simulink model "Hexapod_Robot_Leg"  (Simulink 8.3)
settings: Solver=ode45  StartTime=0.0  StopTime=inf  RelTol=1e-3
undefined symbols (not defined in the file): get, hot
libraries: mblibv1 x70, simulink_need_slupdate x18, vrlib x7, dspsnks4 x1
(part 2 of 2)

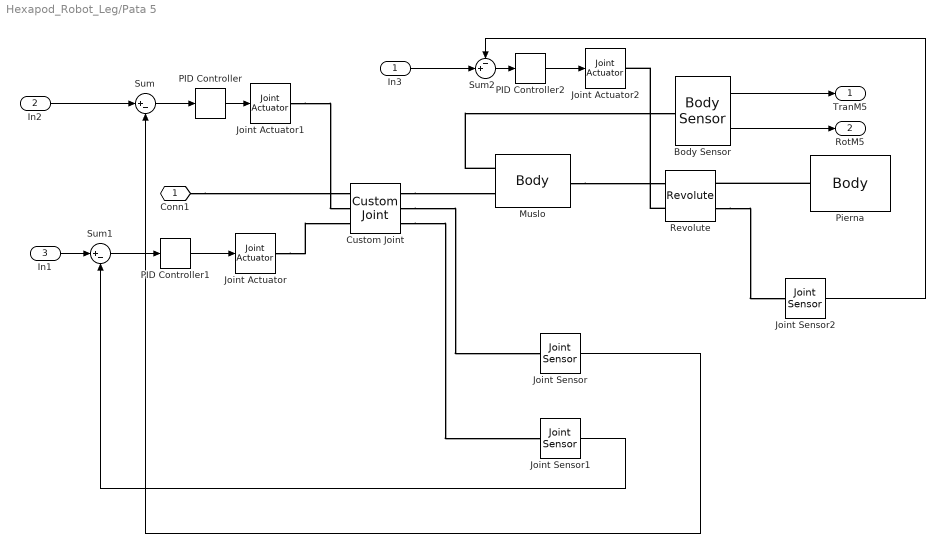
== system Hexapod_Robot_Leg/Pata 5 ==
  In3 : Inport
  In2 : Inport  Port=2
  In1 : Inport  Port=3
  Body Sensor : mblibv1/Sensors &  Actuators/Body Sensor  UpdateFromCAD=off  PhysicalDomain=Mechanical  PortType=blob  Muxed=off  Pose=on  Angle=on  AngleUnits=deg  ArcVelocity=off  ArcVelocityUnits=deg/s  ArcAcceleration=off  ArcAccelerationUnits=deg/s^2  CoordPosition=on  CoordPositionUnits=cm  Velocity=off  VelocityUnits=m/s  Acceleration=off  AccelerationUnits=m/s^2  Quaternion=on  QuaternionDT=off  QuaternionDDT=off  QuaternionUnits=off  OutputVector=[1]  ActiveIO=on  Width=12  DialogClass=MechanicalSensorBlock  ReferenceFrame=Absolute (World)
  Custom Joint : mblibv1/Joints/Custom Joint  LConnTagsString=__newl0|SA1|SA2  RConnTagsString=__newr0|SA1|SA2  UpdateFromCAD=off  NumSAPorts=4  CutJoint=off  MarkAsCut=off  Primitives=prismatic  PrimitiveProps=R1$World$[0 1 0]$revolute#R2$World$[0 0 1]$Revolute  DialogClass=JointBlock  R1Axis=[0 1 0]  R2Axis=[0 0 1]  R3Axis=[]  P1Axis=[]  P2Axis=[]  P3Axis=[]  SAxis=[]
  Joint Actuator : mblibv1/Sensors &  Actuators/Joint Actuator  UpdateFromCAD=off  PhysicalDomain=Mechanical  PortType=blob  ActuationStyle=Force  AngleUnits=deg  ArcVelocityUnits=deg/s  ArcAccelerationUnits=deg/s^2  CoordPositionUnits=m  VelocityUnits=m/s  AccelerationUnits=m/s^2  ForceUnits=N  TorqueUnits=N*m  ActiveIO=on  Width=1  DialogClass=MechanicalActuatorBlock  Primitive=R2  ReferenceFrame=Absolute (World)
  Joint Actuator1 : mblibv1/Sensors &  Actuators/Joint Actuator  UpdateFromCAD=off  PhysicalDomain=Mechanical  PortType=blob  ActuationStyle=Force  AngleUnits=deg  ArcVelocityUnits=deg/s  ArcAccelerationUnits=deg/s^2  CoordPositionUnits=m  VelocityUnits=m/s  AccelerationUnits=m/s^2  ForceUnits=N  TorqueUnits=N*m  ActiveIO=on  Width=1  DialogClass=MechanicalActuatorBlock  Primitive=R1  ReferenceFrame=Absolute (World)
  Joint Actuator2 : mblibv1/Sensors &  Actuators/Joint Actuator  UpdateFromCAD=off  PhysicalDomain=Mechanical  PortType=blob  ActuationStyle=Force  AngleUnits=deg  ArcVelocityUnits=deg/s  ArcAccelerationUnits=deg/s^2  CoordPositionUnits=m  VelocityUnits=m/s  AccelerationUnits=m/s^2  ForceUnits=N  TorqueUnits=N*m  ActiveIO=on  Width=1  DialogClass=MechanicalActuatorBlock  Primitive=R1  ReferenceFrame=Absolute (World)
  Joint Sensor : mblibv1/Sensors &  Actuators/Joint Sensor  UpdateFromCAD=off  PhysicalDomain=Mechanical  PortType=blob  Muxed=on  Pose=off  Angle=on  AngleUnits=deg  ArcVelocity=off  ArcVelocityUnits=deg/s  ArcAcceleration=off  ArcAccelerationUnits=deg/s^2  CoordPosition=on  CoordPositionUnits=m  Velocity=off  VelocityUnits=m/s  Acceleration=off  AccelerationUnits=m/s^2  Quaternion=on  QuaternionDT=off  QuaternionDDT=off  QuaternionUnits=off  OutputVector=[1]  ActiveIO=on  Width=1  DialogClass=MechanicalSensorBlock  Primitive=R1  Force=off  ForceUnits=N  Torque=off  TorqueUnits=N*m  ReferenceFrame=Absolute (World)  ReactionSensedSide=Base  ReactionReferenceFrame=Absolute (World)  ReactionForce=off  ReactionForceUnits=N  ReactionMoment=off  ReactionMomentUnits=N*m
  Joint Sensor1 : mblibv1/Sensors &  Actuators/Joint Sensor  UpdateFromCAD=off  PhysicalDomain=Mechanical  PortType=blob  Muxed=on  Pose=off  Angle=on  AngleUnits=deg  ArcVelocity=off  ArcVelocityUnits=deg/s  ArcAcceleration=off  ArcAccelerationUnits=deg/s^2  CoordPosition=on  CoordPositionUnits=m  Velocity=off  VelocityUnits=m/s  Acceleration=off  AccelerationUnits=m/s^2  Quaternion=on  QuaternionDT=off  QuaternionDDT=off  QuaternionUnits=off  OutputVector=[1]  ActiveIO=on  Width=1  DialogClass=MechanicalSensorBlock  Primitive=R2  Force=off  ForceUnits=N  Torque=off  TorqueUnits=N*m  ReferenceFrame=Absolute (World)  ReactionSensedSide=Base  ReactionReferenceFrame=Absolute (World)  ReactionForce=off  ReactionForceUnits=N  ReactionMoment=off  ReactionMomentUnits=N*m
  Joint Sensor2 : mblibv1/Sensors &  Actuators/Joint Sensor  UpdateFromCAD=off  PhysicalDomain=Mechanical  PortType=blob  Muxed=on  Pose=off  Angle=on  AngleUnits=deg  ArcVelocity=off  ArcVelocityUnits=deg/s  ArcAcceleration=off  ArcAccelerationUnits=deg/s^2  CoordPosition=on  CoordPositionUnits=m  Velocity=off  VelocityUnits=m/s  Acceleration=off  AccelerationUnits=m/s^2  Quaternion=on  QuaternionDT=off  QuaternionDDT=off  QuaternionUnits=off  OutputVector=[1]  ActiveIO=on  Width=1  DialogClass=MechanicalSensorBlock  Primitive=R1  Force=off  ForceUnits=N  Torque=off  TorqueUnits=N*m  ReferenceFrame=Absolute (World)  ReactionSensedSide=Base  ReactionReferenceFrame=Absolute (World)  ReactionForce=off  ReactionForceUnits=N  ReactionMoment=off  ReactionMomentUnits=N*m
  Muslo : mblibv1/Bodies/Body  LConnTagsString=CS3|CS1  RConnTagsString=CS2  UpdateFromCAD=off  DialogClass=MechanicalBodyBlock  Mass=5000  MassUnits=g  InertiaUnits=g*cm^2  Inertia=[197916.6667 0 0;0 197916.6667 0;0 0 15625]  Shape=Cylinder  ShapeDims=[1 1]  ShapeUnits=m  ShapeUse=false  Density=1  DensityUnits=kg/m^3  DensityUse=false  GraphicsMode=MACHINE_DEFAULT  BodyColorSelMode=MACHINE_DEFAULT  BodyColor=[1;0;0]  AttachedToCS=CG  CG=Left$CG$[-5 0 0]$CS1$CS1$cm$[0 0 0]$Euler X-Y-Z$deg$WORLD$false  WorkingFrames=Left$CS3$[0 0 0]$CS1$CS1$cm$[0 0 0]$Euler X-Y-Z$deg$WORLD$true#Left$CS1$[0 0 0]$Adjoining$Adjoining$cm$[0 0 0]$Euler X-Y-Z$deg$WORLD$true#Right$CS2$[-10 0 0]$CS1$CS1$cm$[0 0 0]$Euler X-Y-Z$deg$WORLD$true  CGPos=[-5 0 0]  CGRot=[0 0 0]  CS0Pos=[]  CS0Rot=[]  CS1Pos=[0 0 0]  CS1Rot=[0 0 0]  CS2Pos=[-10 0 0]  CS2Rot=[0 0 0]  CS3Pos=[0 0 0]  CS3Rot=[0 0 0]  CS4Pos=[]  CS4Rot=[]  CS5Pos=[]  CS5Rot=[]  CS6Pos=[]  CS6Rot=[]  CS7Pos=[]  CS7Rot=[]  CS8Pos=[]  CS8Rot=[]  CS9Pos=[]  CS9Rot=[]  CS10Pos=[]  CS10Rot=[]  CS11Pos=[]  CS11Rot=[]  CS12Pos=[]  CS12Rot=[]  CS13Pos=[]  CS13Rot=[]  CS14Pos=[]  CS14Rot=[]  CS15Pos=[]  CS15Rot=[]  CS16Pos=[]  CS16Rot=[]  CS17Pos=[]  CS17Rot=[]  CS18Pos=[]  CS18Rot=[]  CS19Pos=[]  CS19Rot=[]  CS20Pos=[]  CS20Rot=[]
  PID Controller : simulink_need_slupdate/PID Controller  P=10  I=0  D=2
  PID Controller1 : simulink_need_slupdate/PID Controller  P=10  I=0  D=2
  PID Controller2 : simulink_need_slupdate/PID Controller  P=10  I=0  D=2
  Pierna : mblibv1/Bodies/Body  LConnTagsString=CS1  UpdateFromCAD=off  DialogClass=MechanicalBodyBlock  Mass=5000  MassUnits=g  InertiaUnits=g*cm^2  Inertia=[669479.1667 0 0;0 669479.1667 0;0 0 1406.25]  Shape=Cylinder  ShapeDims=[1 1]  ShapeUnits=m  ShapeUse=false  Density=1  DensityUnits=kg/m^3  DensityUse=false  GraphicsMode=MACHINE_DEFAULT  BodyColorSelMode=MACHINE_DEFAULT  BodyColor=[1;0;0]  AttachedToCS=CG  CG=Left$CG$[0 -10 0]$CS1$CS1$cm$[0 0 0]$Euler X-Y-Z$deg$WORLD$false  WorkingFrames=Left$CS1$[0 0 0]$Adjoining$Adjoining$cm$[0 0 0]$Euler X-Y-Z$deg$WORLD$true#Left$CS2$[0 -20 0]$CS1$CS1$cm$[0 0 0]$Euler X-Y-Z$deg$WORLD$false  CGPos=[0 -10 0]  CGRot=[0 0 0]  CS0Pos=[]  CS0Rot=[]  CS1Pos=[0 0 0]  CS1Rot=[0 0 0]  CS2Pos=[0 -20 0]  CS2Rot=[0 0 0]  CS3Pos=[]  CS3Rot=[]  CS4Pos=[]  CS4Rot=[]  CS5Pos=[]  CS5Rot=[]  CS6Pos=[]  CS6Rot=[]  CS7Pos=[]  CS7Rot=[]  CS8Pos=[]  CS8Rot=[]  CS9Pos=[]  CS9Rot=[]  CS10Pos=[]  CS10Rot=[]  CS11Pos=[]  CS11Rot=[]  CS12Pos=[]  CS12Rot=[]  CS13Pos=[]  CS13Rot=[]  CS14Pos=[]  CS14Rot=[]  CS15Pos=[]  CS15Rot=[]  CS16Pos=[]  CS16Rot=[]  CS17Pos=[]  CS17Rot=[]  CS18Pos=[]  CS18Rot=[]  CS19Pos=[]  CS19Rot=[]  CS20Pos=[]  CS20Rot=[]
  Revolute : mblibv1/Joints/Revolute  LConnTagsString=__newl0|SA1  RConnTagsString=__newr0|SA1  UpdateFromCAD=off  NumSAPorts=2  CutJoint=off  MarkAsCut=off  Primitives=prismatic  PrimitiveProps=R1$World$[0 0 1]$revolute  DialogClass=JointBlock  R1Axis=[0 0 1]
  Sum : Sum  Inputs=|+-
  Sum1 : Sum  Inputs=|+-
  Sum2 : Sum  Inputs=-+|
  Conn1 : PMIOPort  Port=1  Side=Left
  TranM5 : Outport
  RotM5 : Outport  Port=2
  wires:
  Joint Sensor/1 -> Sum/2
  Joint Sensor1/1 -> Sum1/2
  Joint Sensor2/1 -> Sum2/1
  PID Controller/1 -> Joint Actuator1/1
  Sum/1 -> PID Controller/1
  In2/1 -> Sum/1
  In1/1 -> Sum1/1
  Sum1/1 -> PID Controller1/1
  PID Controller1/1 -> Joint Actuator/1
  In3/1 -> Sum2/2
  Sum2/1 -> PID Controller2/1
  PID Controller2/1 -> Joint Actuator2/1
  Body Sensor/1 -> TranM5/1
  Body Sensor/2 -> RotM5/1
  connections:
  Revolute/LConn2 -- Joint Actuator2/RConn1
  Revolute/RConn2 -- Joint Sensor2/LConn1
  Muslo/RConn1 -- Revolute/LConn1
  Pierna/LConn1 -- Revolute/RConn1
  Conn1/RConn1 -- Custom Joint/LConn1
  Custom Joint/RConn1 -- Muslo/LConn2
  Joint Actuator1/RConn1 -- Custom Joint/LConn2
  Joint Actuator/RConn1 -- Custom Joint/LConn3
  Custom Joint/RConn2 -- Joint Sensor/LConn1
  Custom Joint/RConn3 -- Joint Sensor1/LConn1
  Muslo/LConn1 -- Body Sensor/LConn1

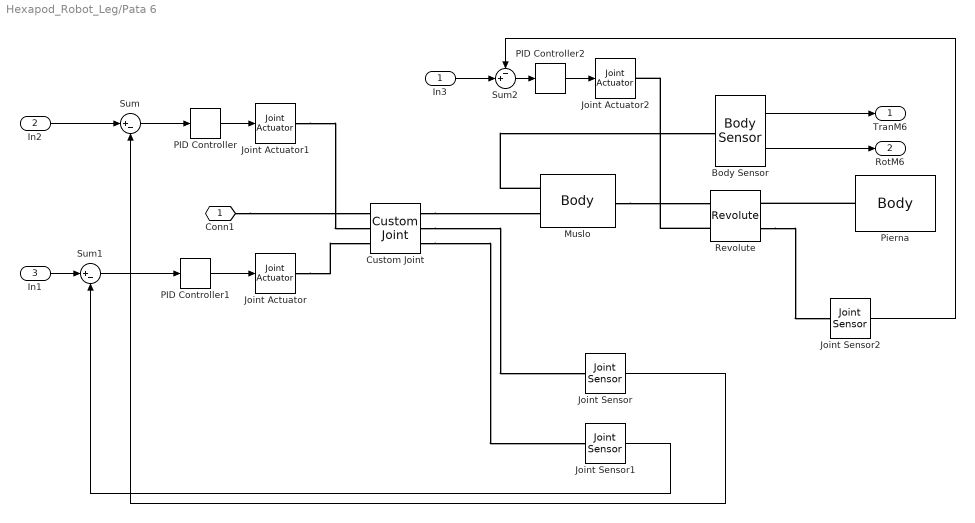
== system Hexapod_Robot_Leg/Pata 6 ==
  In3 : Inport
  In2 : Inport  Port=2
  In1 : Inport  Port=3
  Body Sensor : mblibv1/Sensors &  Actuators/Body Sensor  UpdateFromCAD=off  PhysicalDomain=Mechanical  PortType=blob  Muxed=off  Pose=on  Angle=on  AngleUnits=deg  ArcVelocity=off  ArcVelocityUnits=deg/s  ArcAcceleration=off  ArcAccelerationUnits=deg/s^2  CoordPosition=on  CoordPositionUnits=cm  Velocity=off  VelocityUnits=m/s  Acceleration=off  AccelerationUnits=m/s^2  Quaternion=on  QuaternionDT=off  QuaternionDDT=off  QuaternionUnits=off  OutputVector=[1]  ActiveIO=on  Width=12  DialogClass=MechanicalSensorBlock  ReferenceFrame=Absolute (World)
  Custom Joint : mblibv1/Joints/Custom Joint  LConnTagsString=__newl0|SA1|SA2  RConnTagsString=__newr0|SA1|SA2  UpdateFromCAD=off  NumSAPorts=4  CutJoint=off  MarkAsCut=off  Primitives=prismatic  PrimitiveProps=R1$World$[0 1 0]$revolute#R2$World$[0 0 1]$Revolute  DialogClass=JointBlock  R1Axis=[0 1 0]  R2Axis=[0 0 1]  R3Axis=[]  P1Axis=[]  P2Axis=[]  P3Axis=[]  SAxis=[]
  Joint Actuator : mblibv1/Sensors &  Actuators/Joint Actuator  UpdateFromCAD=off  PhysicalDomain=Mechanical  PortType=blob  ActuationStyle=Force  AngleUnits=deg  ArcVelocityUnits=deg/s  ArcAccelerationUnits=deg/s^2  CoordPositionUnits=m  VelocityUnits=m/s  AccelerationUnits=m/s^2  ForceUnits=N  TorqueUnits=N*m  ActiveIO=on  Width=1  DialogClass=MechanicalActuatorBlock  Primitive=R2  ReferenceFrame=Absolute (World)
  Joint Actuator1 : mblibv1/Sensors &  Actuators/Joint Actuator  UpdateFromCAD=off  PhysicalDomain=Mechanical  PortType=blob  ActuationStyle=Force  AngleUnits=deg  ArcVelocityUnits=deg/s  ArcAccelerationUnits=deg/s^2  CoordPositionUnits=m  VelocityUnits=m/s  AccelerationUnits=m/s^2  ForceUnits=N  TorqueUnits=N*m  ActiveIO=on  Width=1  DialogClass=MechanicalActuatorBlock  Primitive=R1  ReferenceFrame=Absolute (World)
  Joint Actuator2 : mblibv1/Sensors &  Actuators/Joint Actuator  UpdateFromCAD=off  PhysicalDomain=Mechanical  PortType=blob  ActuationStyle=Force  AngleUnits=deg  ArcVelocityUnits=deg/s  ArcAccelerationUnits=deg/s^2  CoordPositionUnits=m  VelocityUnits=m/s  AccelerationUnits=m/s^2  ForceUnits=N  TorqueUnits=N*m  ActiveIO=on  Width=1  DialogClass=MechanicalActuatorBlock  Primitive=R1  ReferenceFrame=Absolute (World)
  Joint Sensor : mblibv1/Sensors &  Actuators/Joint Sensor  UpdateFromCAD=off  PhysicalDomain=Mechanical  PortType=blob  Muxed=on  Pose=off  Angle=on  AngleUnits=deg  ArcVelocity=off  ArcVelocityUnits=deg/s  ArcAcceleration=off  ArcAccelerationUnits=deg/s^2  CoordPosition=on  CoordPositionUnits=m  Velocity=off  VelocityUnits=m/s  Acceleration=off  AccelerationUnits=m/s^2  Quaternion=on  QuaternionDT=off  QuaternionDDT=off  QuaternionUnits=off  OutputVector=[1]  ActiveIO=on  Width=1  DialogClass=MechanicalSensorBlock  Primitive=R1  Force=off  ForceUnits=N  Torque=off  TorqueUnits=N*m  ReferenceFrame=Absolute (World)  ReactionSensedSide=Base  ReactionReferenceFrame=Absolute (World)  ReactionForce=off  ReactionForceUnits=N  ReactionMoment=off  ReactionMomentUnits=N*m
  Joint Sensor1 : mblibv1/Sensors &  Actuators/Joint Sensor  UpdateFromCAD=off  PhysicalDomain=Mechanical  PortType=blob  Muxed=on  Pose=off  Angle=on  AngleUnits=deg  ArcVelocity=off  ArcVelocityUnits=deg/s  ArcAcceleration=off  ArcAccelerationUnits=deg/s^2  CoordPosition=on  CoordPositionUnits=m  Velocity=off  VelocityUnits=m/s  Acceleration=off  AccelerationUnits=m/s^2  Quaternion=on  QuaternionDT=off  QuaternionDDT=off  QuaternionUnits=off  OutputVector=[1]  ActiveIO=on  Width=1  DialogClass=MechanicalSensorBlock  Primitive=R2  Force=off  ForceUnits=N  Torque=off  TorqueUnits=N*m  ReferenceFrame=Absolute (World)  ReactionSensedSide=Base  ReactionReferenceFrame=Absolute (World)  ReactionForce=off  ReactionForceUnits=N  ReactionMoment=off  ReactionMomentUnits=N*m
  Joint Sensor2 : mblibv1/Sensors &  Actuators/Joint Sensor  UpdateFromCAD=off  PhysicalDomain=Mechanical  PortType=blob  Muxed=on  Pose=off  Angle=on  AngleUnits=deg  ArcVelocity=off  ArcVelocityUnits=deg/s  ArcAcceleration=off  ArcAccelerationUnits=deg/s^2  CoordPosition=on  CoordPositionUnits=m  Velocity=off  VelocityUnits=m/s  Acceleration=off  AccelerationUnits=m/s^2  Quaternion=on  QuaternionDT=off  QuaternionDDT=off  QuaternionUnits=off  OutputVector=[1]  ActiveIO=on  Width=1  DialogClass=MechanicalSensorBlock  Primitive=R1  Force=off  ForceUnits=N  Torque=off  TorqueUnits=N*m  ReferenceFrame=Absolute (World)  ReactionSensedSide=Base  ReactionReferenceFrame=Absolute (World)  ReactionForce=off  ReactionForceUnits=N  ReactionMoment=off  ReactionMomentUnits=N*m
  Muslo : mblibv1/Bodies/Body  LConnTagsString=CS3|CS1  RConnTagsString=CS2  UpdateFromCAD=off  DialogClass=MechanicalBodyBlock  Mass=5000  MassUnits=g  InertiaUnits=g*cm^2  Inertia=[197916.6667 0 0;0 197916.6667 0;0 0 15625]  Shape=Cylinder  ShapeDims=[1 1]  ShapeUnits=m  ShapeUse=false  Density=1  DensityUnits=kg/m^3  DensityUse=false  GraphicsMode=MACHINE_DEFAULT  BodyColorSelMode=MACHINE_DEFAULT  BodyColor=[1;0;0]  AttachedToCS=CG  CG="Left$CG$[-5  0 0]$CS1$CS1$cm$[0 0 0]$Euler X-Y-Z$deg$WORLD$false"  WorkingFrames="Left$CS3$[0  0 0]$CS1$CS1$cm$[0 0 0]$Euler X-Y-Z$deg$WORLD$true#Left$CS1$[0 0 0]$Adjoining$Adjoining$cm$[0 0 0]$Euler X-Y-Z$deg$WORLD$true#Right$CS2$[-10 0 0]$CS1$CS1$cm$[0 0 0]$Euler X-Y-Z$deg$WORLD$true"  CGPos="[-5  0 0]"  CGRot=[0 0 0]  CS0Pos=[]  CS0Rot=[]  CS1Pos=[0 0 0]  CS1Rot=[0 0 0]  CS2Pos=[-10 0 0]  CS2Rot=[0 0 0]  CS3Pos="[0  0 0]"  CS3Rot=[0 0 0]  CS4Pos=[]  CS4Rot=[]  CS5Pos=[]  CS5Rot=[]  CS6Pos=[]  CS6Rot=[]  CS7Pos=[]  CS7Rot=[]  CS8Pos=[]  CS8Rot=[]  CS9Pos=[]  CS9Rot=[]  CS10Pos=[]  CS10Rot=[]  CS11Pos=[]  CS11Rot=[]  CS12Pos=[]  CS12Rot=[]  CS13Pos=[]  CS13Rot=[]  CS14Pos=[]  CS14Rot=[]  CS15Pos=[]  CS15Rot=[]  CS16Pos=[]  CS16Rot=[]  CS17Pos=[]  CS17Rot=[]  CS18Pos=[]  CS18Rot=[]  CS19Pos=[]  CS19Rot=[]  CS20Pos=[]  CS20Rot=[]
  PID Controller : simulink_need_slupdate/PID Controller  P=10  I=0  D=2
  PID Controller1 : simulink_need_slupdate/PID Controller  P=10  I=0  D=2
  PID Controller2 : simulink_need_slupdate/PID Controller  P=10  I=0  D=2
  Pierna : mblibv1/Bodies/Body  LConnTagsString=CS1  UpdateFromCAD=off  DialogClass=MechanicalBodyBlock  Mass=5000  MassUnits=g  InertiaUnits=g*cm^2  Inertia=[669479.1667 0 0;0 669479.1667 0;0 0 1406.25]  Shape=Cylinder  ShapeDims=[1 1]  ShapeUnits=m  ShapeUse=false  Density=1  DensityUnits=kg/m^3  DensityUse=false  GraphicsMode=MACHINE_DEFAULT  BodyColorSelMode=MACHINE_DEFAULT  BodyColor=[1;0;0]  AttachedToCS=CG  CG=Left$CG$[0 -10 0]$CS1$CS1$cm$[0 0 0]$Euler X-Y-Z$deg$WORLD$false  WorkingFrames=Left$CS1$[0 0 0]$Adjoining$Adjoining$cm$[0 0 0]$Euler X-Y-Z$deg$WORLD$true#Left$CS2$[0 -20 0]$CS1$CS1$cm$[0 0 0]$Euler X-Y-Z$deg$WORLD$false  CGPos=[0 -10 0]  CGRot=[0 0 0]  CS0Pos=[]  CS0Rot=[]  CS1Pos=[0 0 0]  CS1Rot=[0 0 0]  CS2Pos=[0 -20 0]  CS2Rot=[0 0 0]  CS3Pos=[]  CS3Rot=[]  CS4Pos=[]  CS4Rot=[]  CS5Pos=[]  CS5Rot=[]  CS6Pos=[]  CS6Rot=[]  CS7Pos=[]  CS7Rot=[]  CS8Pos=[]  CS8Rot=[]  CS9Pos=[]  CS9Rot=[]  CS10Pos=[]  CS10Rot=[]  CS11Pos=[]  CS11Rot=[]  CS12Pos=[]  CS12Rot=[]  CS13Pos=[]  CS13Rot=[]  CS14Pos=[]  CS14Rot=[]  CS15Pos=[]  CS15Rot=[]  CS16Pos=[]  CS16Rot=[]  CS17Pos=[]  CS17Rot=[]  CS18Pos=[]  CS18Rot=[]  CS19Pos=[]  CS19Rot=[]  CS20Pos=[]  CS20Rot=[]
  Revolute : mblibv1/Joints/Revolute  LConnTagsString=__newl0|SA1  RConnTagsString=__newr0|SA1  UpdateFromCAD=off  NumSAPorts=2  CutJoint=off  MarkAsCut=off  Primitives=prismatic  PrimitiveProps=R1$World$[0 0 1]$revolute  DialogClass=JointBlock  R1Axis=[0 0 1]
  Sum : Sum  Inputs=|+-
  Sum1 : Sum  Inputs=|+-
  Sum2 : Sum  Inputs=-+|
  Conn1 : PMIOPort  Port=1  Side=Left
  TranM6 : Outport
  RotM6 : Outport  Port=2
  wires:
  Joint Sensor/1 -> Sum/2
  Joint Sensor1/1 -> Sum1/2
  Joint Sensor2/1 -> Sum2/1
  PID Controller/1 -> Joint Actuator1/1
  Sum/1 -> PID Controller/1
  In2/1 -> Sum/1
  In1/1 -> Sum1/1
  Sum1/1 -> PID Controller1/1
  PID Controller1/1 -> Joint Actuator/1
  In3/1 -> Sum2/2
  Sum2/1 -> PID Controller2/1
  PID Controller2/1 -> Joint Actuator2/1
  Body Sensor/1 -> TranM6/1
  Body Sensor/2 -> RotM6/1
  connections:
  Revolute/LConn2 -- Joint Actuator2/RConn1
  Revolute/RConn2 -- Joint Sensor2/LConn1
  Muslo/RConn1 -- Revolute/LConn1
  Pierna/LConn1 -- Revolute/RConn1
  Conn1/RConn1 -- Custom Joint/LConn1
  Custom Joint/RConn1 -- Muslo/LConn2
  Joint Actuator1/RConn1 -- Custom Joint/LConn2
  Joint Actuator/RConn1 -- Custom Joint/LConn3
  Custom Joint/RConn2 -- Joint Sensor/LConn1
  Custom Joint/RConn3 -- Joint Sensor1/LConn1
  Muslo/LConn1 -- Body Sensor/LConn1

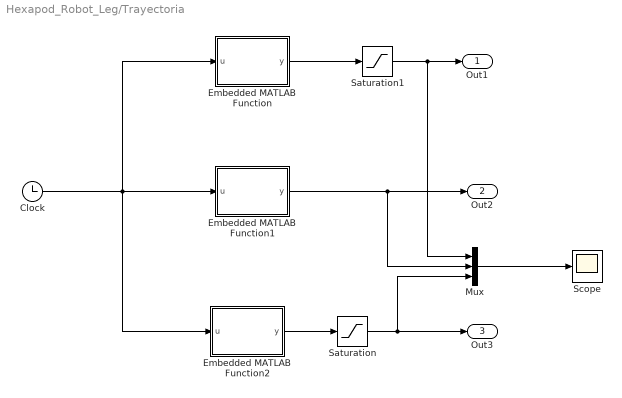
== system Hexapod_Robot_Leg/Trayectoria ==
  Clock : Clock
  Embedded MATLAB Function : MATLAB Function  TreatAsAtomicUnit=on
  Embedded MATLAB Function1 : MATLAB Function  TreatAsAtomicUnit=on
  Embedded MATLAB Function2 : MATLAB Function  TreatAsAtomicUnit=on
  Mux : Mux  Inputs=3
  Saturation : Saturate  UpperLimit=30  LowerLimit=0
  Saturation1 : Saturate  UpperLimit=30  LowerLimit=0
  Scope : Scope
      settings: SaveName=ScopeData2
  Out1 : Outport
  Out2 : Outport  Port=2
  Out3 : Outport  Port=3
  wires:
  Embedded MATLAB Function/1(y) -> Saturation1/1
  Embedded MATLAB Function2/1(y) -> Saturation/1
  Clock/1 -> Embedded MATLAB Function1/1(u), Embedded MATLAB Function/1(u), Embedded MATLAB Function2/1(u)
  Embedded MATLAB Function1/1(y) -> Out2/1, Mux/2
  Saturation/1 -> Out3/1, Mux/3
  Saturation1/1 -> Out1/1, Mux/1
  Mux/1 -> Scope/1

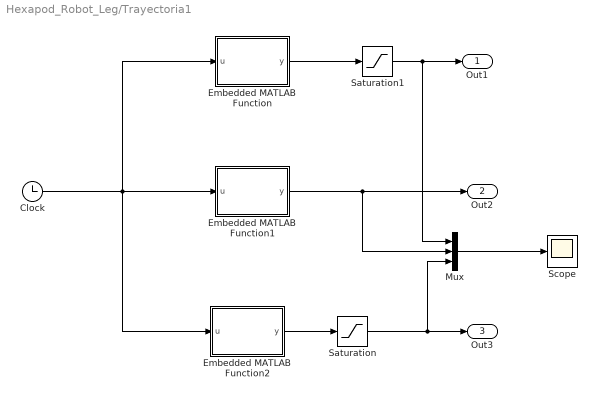
== system Hexapod_Robot_Leg/Trayectoria1 ==
  Clock : Clock
  Embedded MATLAB Function : MATLAB Function  TreatAsAtomicUnit=on
  Embedded MATLAB Function1 : MATLAB Function  TreatAsAtomicUnit=on
  Embedded MATLAB Function2 : MATLAB Function  TreatAsAtomicUnit=on
  Mux : Mux  Inputs=3
  Saturation : Saturate  UpperLimit=30  LowerLimit=0
  Saturation1 : Saturate  UpperLimit=30  LowerLimit=0
  Scope : Scope
  Out1 : Outport
  Out2 : Outport  Port=2
  Out3 : Outport  Port=3
  wires:
  Saturation1/1 -> Out1/1, Mux/1
  Saturation/1 -> Out3/1, Mux/3
  Embedded MATLAB Function1/1(y) -> Out2/1, Mux/2
  Clock/1 -> Embedded MATLAB Function2/1(u), Embedded MATLAB Function/1(u), Embedded MATLAB Function1/1(u)
  Embedded MATLAB Function2/1(y) -> Saturation/1
  Embedded MATLAB Function/1(y) -> Saturation1/1
  Mux/1 -> Scope/1

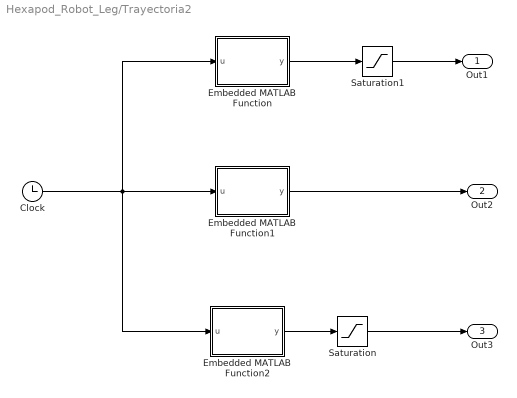
== system Hexapod_Robot_Leg/Trayectoria2 ==
  Clock : Clock
  Embedded MATLAB Function : MATLAB Function  TreatAsAtomicUnit=on
  Embedded MATLAB Function1 : MATLAB Function  TreatAsAtomicUnit=on
  Embedded MATLAB Function2 : MATLAB Function  TreatAsAtomicUnit=on
  Saturation : Saturate  UpperLimit=30  LowerLimit=0
  Saturation1 : Saturate  UpperLimit=30  LowerLimit=0
  Out1 : Outport
  Out2 : Outport  Port=2
  Out3 : Outport  Port=3
  wires:
  Embedded MATLAB Function/1(y) -> Saturation1/1
  Embedded MATLAB Function2/1(y) -> Saturation/1
  Clock/1 -> Embedded MATLAB Function1/1(u), Embedded MATLAB Function/1(u), Embedded MATLAB Function2/1(u)
  Embedded MATLAB Function1/1(y) -> Out2/1
  Saturation/1 -> Out3/1
  Saturation1/1 -> Out1/1

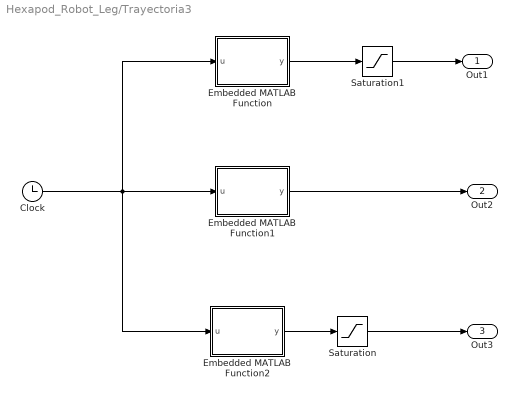
== system Hexapod_Robot_Leg/Trayectoria3 ==
  Clock : Clock
  Embedded MATLAB Function : MATLAB Function  TreatAsAtomicUnit=on
  Embedded MATLAB Function1 : MATLAB Function  TreatAsAtomicUnit=on
  Embedded MATLAB Function2 : MATLAB Function  TreatAsAtomicUnit=on
  Saturation : Saturate  UpperLimit=30  LowerLimit=0
  Saturation1 : Saturate  UpperLimit=30  LowerLimit=0
  Out1 : Outport
  Out2 : Outport  Port=2
  Out3 : Outport  Port=3
  wires:
  Saturation1/1 -> Out1/1
  Saturation/1 -> Out3/1
  Embedded MATLAB Function1/1(y) -> Out2/1
  Clock/1 -> Embedded MATLAB Function2/1(u), Embedded MATLAB Function/1(u), Embedded MATLAB Function1/1(u)
  Embedded MATLAB Function2/1(y) -> Saturation/1
  Embedded MATLAB Function/1(y) -> Saturation1/1

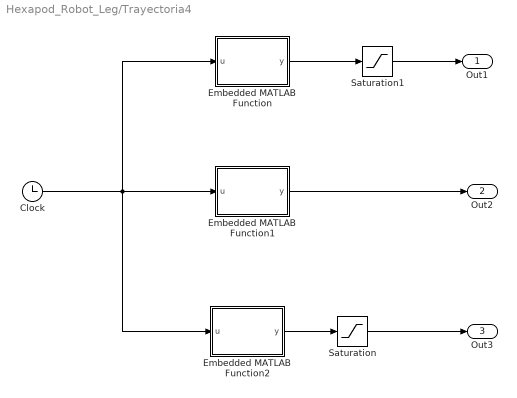
== system Hexapod_Robot_Leg/Trayectoria4 ==
  Clock : Clock
  Embedded MATLAB Function : MATLAB Function  TreatAsAtomicUnit=on
  Embedded MATLAB Function1 : MATLAB Function  TreatAsAtomicUnit=on
  Embedded MATLAB Function2 : MATLAB Function  TreatAsAtomicUnit=on
  Saturation : Saturate  UpperLimit=30  LowerLimit=0
  Saturation1 : Saturate  UpperLimit=30  LowerLimit=0
  Out1 : Outport
  Out2 : Outport  Port=2
  Out3 : Outport  Port=3
  wires:
  Embedded MATLAB Function/1(y) -> Saturation1/1
  Embedded MATLAB Function2/1(y) -> Saturation/1
  Clock/1 -> Embedded MATLAB Function1/1(u), Embedded MATLAB Function/1(u), Embedded MATLAB Function2/1(u)
  Embedded MATLAB Function1/1(y) -> Out2/1
  Saturation/1 -> Out3/1
  Saturation1/1 -> Out1/1

== system Hexapod_Robot_Leg/Trayectoria5 ==
  Clock : Clock
  Embedded MATLAB Function : MATLAB Function  TreatAsAtomicUnit=on
  Embedded MATLAB Function1 : MATLAB Function  TreatAsAtomicUnit=on
  Embedded MATLAB Function2 : MATLAB Function  TreatAsAtomicUnit=on
  Saturation : Saturate  UpperLimit=30  LowerLimit=0
  Saturation1 : Saturate  UpperLimit=30  LowerLimit=0
  Out1 : Outport
  Out2 : Outport  Port=2
  Out3 : Outport  Port=3
  wires:
  Saturation1/1 -> Out1/1
  Saturation/1 -> Out3/1
  Embedded MATLAB Function1/1(y) -> Out2/1
  Clock/1 -> Embedded MATLAB Function2/1(u), Embedded MATLAB Function/1(u), Embedded MATLAB Function1/1(u)
  Embedded MATLAB Function2/1(y) -> Saturation/1
  Embedded MATLAB Function/1(y) -> Saturation1/1

== matlab function Trayectoria/Embedded MATLAB Function1 ==
  data: u input double; y output double
function y = fcn(u)
% This block supports the Embedded MATLAB subset.
% See the help menu for details. 

%angulo theta1 en torno al eje y

y = 50*sin(u);

== matlab function Trayectoria/Embedded MATLAB Function ==
  data: u input double; y output double
function y = fcn(u)
% This block supports the Embedded MATLAB subset.
% See the help menu for details. 
%angulo theta3, entre muslo y pierna

y = 0;   %30*cos(u);

== matlab function Trayectoria/Embedded MATLAB Function2 ==
  data: u input double; y output double
function y = fcn(u)
% This block supports the Embedded MATLAB subset.
% See the help menu for details. 

%angulo theta2 en torno al eje x

y = 30*sin(u - pi/2);

== matlab function Trayectoria1/Embedded MATLAB Function ==
  data: u input double; y output double
function y = fcn(u)
% This block supports the Embedded MATLAB subset.
% See the help menu for details. 
%angulo theta3, entre muslo y pierna

y = 0;  %30*cos(u);

== matlab function Trayectoria1/Embedded MATLAB Function1 ==
  data: u input double; y output double
function y = fcn(u)
% This block supports the Embedded MATLAB subset.
% See the help menu for details. 

%angulo theta1 en torno al eje y

y = -50*sin(u);

== matlab function Trayectoria1/Embedded MATLAB Function2 ==
  data: u input double; y output double
function y = fcn(u)
% This block supports the Embedded MATLAB subset.
% See the help menu for details. 

%angulo theta2 en torno al eje x

y = 30*cos(u);

== matlab function Trayectoria2/Embedded MATLAB Function ==
  data: u input double; y output double
function y = fcn(u)
% This block supports the Embedded MATLAB subset.
% See the help menu for details. 
%angulo theta3, entre muslo y pierna

y = 0;  %30*cos(u);

== matlab function Trayectoria2/Embedded MATLAB Function1 ==
  data: u input double; y output double
function y = fcn(u)
% This block supports the Embedded MATLAB subset.
% See the help menu for details. 

%angulo theta1 en torno al eje y

y = 50*sin(u);

== matlab function Trayectoria2/Embedded MATLAB Function2 ==
  data: u input double; y output double
function y = fcn(u)
% This block supports the Embedded MATLAB subset.
% See the help menu for details. 

%angulo theta2 en torno al eje x

y = 30*sin(u-pi/2);

== matlab function Trayectoria3/Embedded MATLAB Function ==
  data: u input double; y output double
function y = fcn(u)
% This block supports the Embedded MATLAB subset.
% See the help menu for details. 
%angulo theta3, entre muslo y pierna

y = 0;  %30*cos(u);

== matlab function Trayectoria3/Embedded MATLAB Function1 ==
  data: u input double; y output double
function y = fcn(u)
% This block supports the Embedded MATLAB subset.
% See the help menu for details. 

%angulo theta1 en torno al eje y

y = -50*sin(u);

== matlab function Trayectoria3/Embedded MATLAB Function2 ==
  data: u input double; y output double
function y = fcn(u)
% This block supports the Embedded MATLAB subset.
% See the help menu for details. 

%angulo theta2 en torno al eje x

y = 30*cos(u);

== matlab function Trayectoria4/Embedded MATLAB Function ==
  data: u input double; y output double
function y = fcn(u)
% This block supports the Embedded MATLAB subset.
% See the help menu for details. 
%angulo theta3, entre muslo y pierna

y = 0;  %30*cos(u);

== matlab function Trayectoria4/Embedded MATLAB Function1 ==
  data: u input double; y output double
function y = fcn(u)
% This block supports the Embedded MATLAB subset.
% See the help menu for details. 

%angulo theta1 en torno al eje y

y = 50*sin(u);

== matlab function Trayectoria4/Embedded MATLAB Function2 ==
  data: u input double; y output double
function y = fcn(u)
% This block supports the Embedded MATLAB subset.
% See the help menu for details. 

%angulo theta2 en torno al eje x

y = 30*sin(u - pi/2);

== matlab function Trayectoria5/Embedded MATLAB Function ==
  data: u input double; y output double
function y = fcn(u)
% This block supports the Embedded MATLAB subset.
% See the help menu for details. 
%angulo theta3, entre muslo y pierna

y = 0;  %30*cos(u);

== matlab function Trayectoria5/Embedded MATLAB Function1 ==
  data: u input double; y output double
function y = fcn(u)
% This block supports the Embedded MATLAB subset.
% See the help menu for details. 

%angulo theta1 en torno al eje y

y = -50*sin(u);

== matlab function Trayectoria5/Embedded MATLAB Function2 ==
  data: u input double; y output double
function y = fcn(u)
% This block supports the Embedded MATLAB subset.
% See the help menu for details. 

%angulo theta2 en torno al eje x

y = 30*cos(u);
